simulink model "example_of_convert_spead"  (R2021a)
settings: Solver=VariableStepAuto  StartTime=0.0  StopTime=10.0  RelTol=1e-3
settings Model: Creator=YasserNet  LastModifiedBy=YasserNet

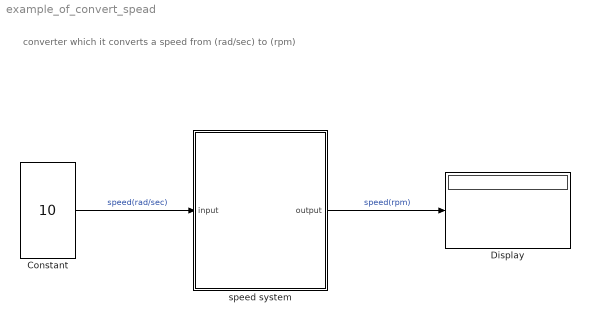
== system example_of_convert_spead ==
  note: converter which it converts a speed from (rad/sec) to (rpm)
  Constant : Constant  Value=10
  Display : Display
  speed system : Subsystem
  wires:
  Constant/1 -> speed system/1(input)  "speed(rad/sec)"
  speed system/1(output) -> Display/1  "speed(rpm)"

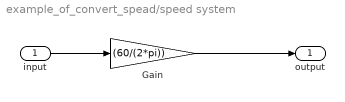
== system example_of_convert_spead/speed system ==
  input : Inport
  Gain : Gain  Gain=(60/(2*pi))
  output : Outport
  wires:
  Gain/1 -> output/1
  input/1 -> Gain/1
